simulink model "dervtv_control_pole_placement"  (R2022b)
settings: Solver=VariableStepAuto  StartTime=0.0  StopTime=10  RelTol=1e-3
values from neighbouring files (symbols this model uses):
  A = [0 1; 0 -1/Tau]    [MPCsys_obs.m]    (also in derivative_control_LQ.m = [0 1; 0 -1/tau]; derivative_control_pole_placement.m = [0 1; 0 -1/tau])
  B = [0 K/Tau]'    [MPCsys_obs.m]    (also in derivative_control_LQ.m = [0 K/tau]'; derivative_control_pole_placement.m = [0 K/tau]')
  C = [1 0]    [MPCsys_obs.m]    (also in derivative_control_LQ.m; derivative_control_pole_placement.m)
  D = 0    [MPCsys_obs.m]    (also in derivative_control_LQ.m; derivative_control_pole_placement.m)
  K_v = K_eng(:, n+1:end)    [derivative_control_pole_placement.m]    (also in luemberger_control_pole_placement.m)
  K_x = K_eng(:, 1:n)    [derivative_control_pole_placement.m]    (also in luemberger_control_pole_placement.m)
settings Model: Creator=Davvy  LastModifiedBy=Davvy

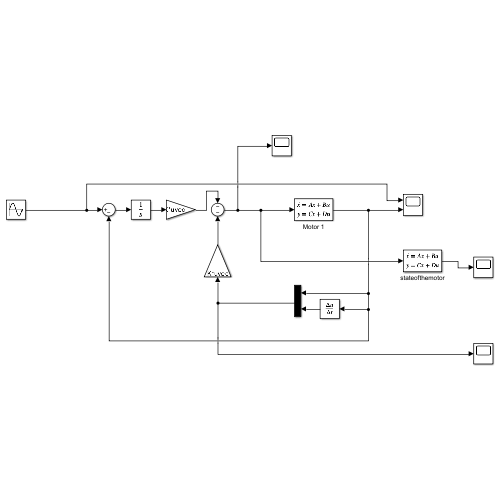
[thumbnail: Simulink's stored preview of the top-level diagram]
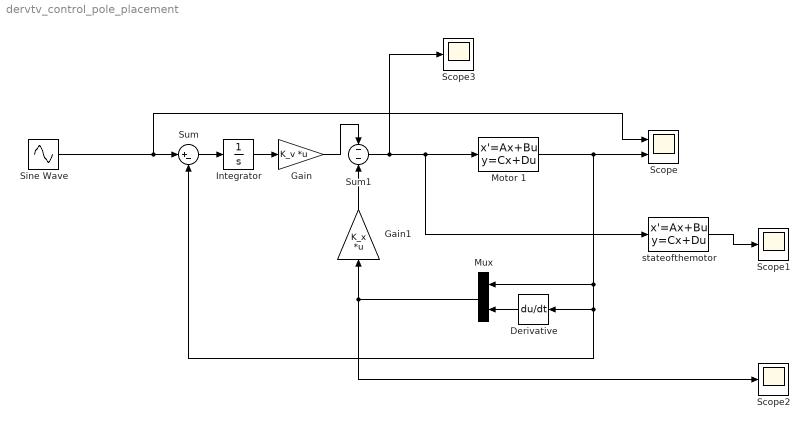
== system dervtv_control_pole_placement ==
  Derivative : Derivative
  Gain : Gain  Gain=K_v  Multiplication=Matrix(K*u) (u vector)
  Gain1 : Gain  Gain=K_x  Multiplication=Matrix(K*u) (u vector)
  Integrator : Integrator
  Motor 1 : StateSpace  A=A  B=B  C=C  D=D  InitialCondition=0
  Mux : Mux  Inputs=2
  Scope : Scope  NumInputPorts=2
  Scope1 : Scope
  Scope2 : Scope
  Scope3 : Scope
  Sine Wave : Sin  Frequency=14  SampleTime=0
  Sum : Sum  Inputs=|+-
  Sum1 : Sum  Inputs=--
  stateofthemotor : StateSpace  A=A  B=B  C=eye(2)  D=[0;0]  InitialCondition=0
  wires:
  Sine Wave/1 -> Scope/1, Sum/1
  Mux/1 -> Scope2/1, Gain1/1
  Gain1/1 -> Sum1/2
  Sum1/1 -> Scope3/1, stateofthemotor/1, Motor 1/1
  Gain/1 -> Sum1/1
  Sum/1 -> Integrator/1
  Integrator/1 -> Gain/1
  stateofthemotor/1 -> Scope1/1
  Motor 1/1 -> Mux/1, Derivative/1, Sum/2, Scope/2
  Derivative/1 -> Mux/2
